simulink model "PubIfDecisionTOS_MDL"  (R2020b)
settings: configuration reference "DspaceConfig" (kept outside this file)
PostLoadFcn:
  | if any(exist('dsrtsu_mdlpostloadfcn', 'file') ~= 0), dsrtsu_mdlpostloadfcn('Execute', bdroot); end
InitFcn:
  | , if any(exist('dsmpb_private', 'file') ~= 0), dsmpb_private('dsmpb_mdlclblib', 'Init', bdroot); end,
undefined symbols (not defined in the file or in its folder): C_TOS_ACCEgoRAxletoFbumplength_m, C_TOS_ACCTargetFront_Flag, C_TOS_AEBJAPedObjDxThre_Val, C_TOS_AEBJAPedObjDyThre_Val, C_TOS_AEBJATargetSize_Val, C_TOS_AEBJAVehObjDxThre_Val, C_TOS_AEBJAVehObjDyThre_Val, C_TOS_AEBJuncPedTargetSize_Val, C_TOS_AEBLatObjDxThre_Val, C_TOS_AEBLatPedDyThre_Val, C_TOS_AEBLatTargetSize_Val, C_TOS_AEBLongTargetInEgoFront_Flag, C_TOS_axAbsGround_Parameter, C_TOS_CameraConfirmedFlag, C_TOS_CNsubjWidth, C_TOS_CurrentLaneCoreMinWidth_Val, C_TOS_CutInProb_Val_Zero, C_TOS_CutOutProb_Val_Zero, C_TOS_D2R_Val, C_TOS_DefaultValueObjectToCenterLine_dy, C_TOS_EgoCarWidth_Val, C_TOS_EgoDxRefPoint_m, C_TOS_EgoRAxletoFbumplength_m, C_TOS_HalfWidthVehicle_Con, C_TOS_HWA_CurrentLaneFlag, C_TOS_HWA_LeftLaneFlag, C_TOS_HWA_MovingDir_Vaild, C_TOS_HWA_MovState_Vaild, C_TOS_HWA_RightLaneFlag, C_TOS_LaneLineCourseErrorFront, C_TOS_LaneLineCourseErrorRear, C_TOS_MotorbikeDefaultWidth_m, C_TOS_NumberOfEffectiveTargets, C_TOS_Obj_Age_Val, C_TOS_Objdx_Constraint_Val, C_TOS_ObjectDefaultWidth_m, C_TOS_ObjInCurrentLane_Val, C_TOS_ObjInCurrentLaneValid, C_TOS_ObjInLeftLaneValid, C_TOS_ObjInRightLaneValid, C_TOS_ObjNotInCurrentLane_Val, C_TOS_ObjNotREElementType, C_TOS_ObjPredictDis_dy_ConstantVal_Zeros, C_TOS_ObjToCenterLine_ConstantVal_Zeros, C_TOS_OFMObjIDInvilad_Val, C_TOS_PIL_LatDisCons_Val_zero, C_TOS_PIL_ObjectCutInFlag_b, C_TOS_PIL_ObjectCutOutFlag_b, C_TOS_PIL_ObjLaneProb_al_Val, C_TOS_PP_ObjFusType_FC_Confirm_b, C_TOS_PP_ObjFusType_FC_FR_Confirm_b, C_TOS_PP_ObjFusType_FR_Confirm_b, C_TOS_RE_80BoolDefault_Val, C_TOS_RE_80Single181Default_Val, C_TOS_RE_80Single255Default_Val, C_TOS_RE_80Uint8Default_Val, C_TOS_RE_D2R, C_TOS_RE_D_180_Val, C_TOS_RE_InvalidObjectID_Val, C_TOS_RE_InvalidTargetChainDir_Val ... (+142)
libraries: simulink x1650, TOS_LIB x361, canfdmsglib x14
(part 58 of 69)

== system PubIfDecisionTOS_MDL/TOS_20201112/TOS_2012080320/TOS/AEB/TOS_AEBLong/AEBLong_Confirm/AEBLong/AEBLong_TrgConfirm/AEBLongTrgJudg/TOS_AEBLong_TargetMovingDir/ObjMovingDirSignalProcessing1/ObjMovingDirSignalProcessing2 ==
  note: fun2:目标运动方向处理 (ACC/AEB/HWA_LC/ELK/LCKie)
  PP_OncomingMovingDirFlg : Inport
  PP_CrossingMovingDirFlg : Inport  Port=2
  Object_MovingOrientation : Inport  Port=3
  Object_HeadingAngle : Inport  Port=4
  Abs : Abs
  Compare To Constant : simulink/Logic and Bit Operations/Compare To Constant  relop===  const=OFM_OBJ_ORIENTATION_E.NORTH  OutDataTypeStr=boolean
      settings: AttributesFormatString=OFM_OBJ_ORIENTATION_E.NORTH = 9
  Compare To Constant1 : simulink/Logic and Bit Operations/Compare To Constant  relop=>=  const=P_TOS_ObjInSameDirYawAngMinThre_Val  OutDataTypeStr=boolean
      settings: AttributesFormatString=P_TOS_ObjInSameDirYawAngMinThre_Val = 0
  Compare To Constant2 : simulink/Logic and Bit Operations/Compare To Constant  relop=<=  const=P_TOS_ObjInSameDirYawAngMaxThre_Val  OutDataTypeStr=boolean
      settings: AttributesFormatString=P_TOS_ObjInSameDirYawAngMaxThre_Val = 45
  Compare To Constant3 : simulink/Logic and Bit Operations/Compare To Constant  relop===  const=OFM_OBJ_ORIENTATION_E.SOUTH  OutDataTypeStr=boolean
      settings: AttributesFormatString=OFM_OBJ_ORIENTATION_E.SOUTH = 5
  Compare To Constant4 : simulink/Logic and Bit Operations/Compare To Constant  relop===  const=OFM_OBJ_ORIENTATION_E.WEST  OutDataTypeStr=boolean
      settings: AttributesFormatString=OFM_OBJ_ORIENTATION_E.WEST = 7
  Compare To Constant5 : simulink/Logic and Bit Operations/Compare To Constant  relop===  const=OFM_OBJ_ORIENTATION_E.EAST  OutDataTypeStr=boolean
      settings: AttributesFormatString=OFM_OBJ_ORIENTATION_E.EAST = 3
  Compare To Constant6 : simulink/Logic and Bit Operations/Compare To Constant  relop=>=  const=P_TOS_ObjLatCroYawAngMaxThre_Val  OutDataTypeStr=boolean
      settings: AttributesFormatString=P_TOS_ObjLatCroYawAngMaxThre_Val = 135
  Compare To Constant7 : simulink/Logic and Bit Operations/Compare To Constant  relop=<=  const=P_TOS_ObjOncomingYawAngMaxThre_Val  OutDataTypeStr=boolean
      settings: AttributesFormatString=P_TOS_ObjOncomingYawAngMaxThre_Val = 180
  Compare To Constant8 : simulink/Logic and Bit Operations/Compare To Constant  relop=>=  const=P_TOS_ObjLatCroYawAngMinThre_Val  OutDataTypeStr=boolean
      settings: AttributesFormatString=P_TOS_ObjLatCroYawAngMinThre_Val = 45
  Compare To Constant9 : simulink/Logic and Bit Operations/Compare To Constant  relop=<=  const=P_TOS_ObjLatCroYawAngMaxThre_Val  OutDataTypeStr=boolean
      settings: AttributesFormatString=P_TOS_ObjLatCroYawAngMaxThre_Val = 135
  Data Type Conversion1 : DataTypeConversion  OutDataTypeStr=uint8
  Data Type Conversion2 : DataTypeConversion  OutDataTypeStr=Enum: OFM_OBJ_ORIENTATION_E
  Enumerated Constant4 : simulink/Sources/Enumerated Constant  OutDataTypeStr=Enum: ObjectMovingOrientation_E  Value=ObjectMovingOrientation_E.SameDir  SampleTime=inf
      settings: AttributesFormatString=ObjectMovingOrientation_E.SameDir = 1
  Enumerated Constant5 : simulink/Sources/Enumerated Constant  OutDataTypeStr=Enum: ObjectMovingOrientation_E  Value=ObjectMovingOrientation_E.OnComingDir  SampleTime=inf
      settings: AttributesFormatString=ObjectMovingOrientation_E.OnComingDir = 2
  Enumerated Constant6 : simulink/Sources/Enumerated Constant  OutDataTypeStr=Enum: ObjectMovingOrientation_E  Value=ObjectMovingOrientation_E.Crossing  SampleTime=inf
      settings: AttributesFormatString=ObjectMovingOrientation_E.Crossing = 3
  Enumerated Constant7 : simulink/Sources/Enumerated Constant  OutDataTypeStr=Enum: ObjectMovingOrientation_E  Value=ObjectMovingOrientation_E.UnknownDir  SampleTime=inf
      settings: AttributesFormatString=ObjectMovingOrientation_E.UnknownDir = 0
  Logical Operator{7..10,13,15} (6 alike) : Logic  Operator=OR  AllPortsSameDT=off  OutDataTypeStr=boolean
  Logical Operator11 : Logic  AllPortsSameDT=off  OutDataTypeStr=boolean
  Logical Operator12 : Logic  AllPortsSameDT=off  OutDataTypeStr=boolean
  Logical Operator14 : Logic  AllPortsSameDT=off  OutDataTypeStr=boolean
  Switch3 : Switch  Criteria=u2 ~= 0
  Switch4 : Switch  Criteria=u2 ~= 0
  Switch5 : Switch  Criteria=u2 ~= 0
  PP_ObjMovingDirSignalProcessing : Outport
  wires:
  Data Type Conversion1/1 -> PP_ObjMovingDirSignalProcessing/1
  Object_MovingOrientation/1 -> Data Type Conversion2/1
  Object_HeadingAngle/1 -> Abs/1
  Logical Operator10/1 -> Logical Operator7/1
  PP_OncomingMovingDirFlg/1 -> [PP_OncomingMovingDirFlg]
  PP_CrossingMovingDirFlg/1 -> [PP_CrossingMovingDirFlg]
  [PP_OncomingMovingDirFlg] -> Logical Operator7/2
  [PP_CrossingMovingDirFlg] -> Logical Operator8/2
  Logical Operator14/1 -> Logical Operator13/2  "ObjLatCrossDirYawValid"
  Enumerated Constant6/1 -> Switch5/1
  Logical Operator12/1 -> Logical Operator9/2
  Compare To Constant6/1 -> Logical Operator11/1
  Compare To Constant1/1 -> Logical Operator12/1
  Enumerated Constant4/1 -> Switch3/1
  Logical Operator7/1 -> Switch4/2
  Logical Operator15/1 -> Logical Operator13/1
  Compare To Constant8/1 -> Logical Operator14/1
  Compare To Constant7/1 -> Logical Operator11/2
  Compare To Constant3/1 -> Logical Operator10/1
  Switch4/1 -> Switch5/3
  Logical Operator11/1 -> Logical Operator10/2
  Compare To Constant4/1 -> Logical Operator15/1
  Compare To Constant5/1 -> Logical Operator15/2
  Compare To Constant2/1 -> Logical Operator12/2
  Compare To Constant9/1 -> Logical Operator14/2
  Logical Operator9/1 -> Switch3/2
  Logical Operator8/1 -> Switch5/2
  Abs/1 -> Compare To Constant7/1, Compare To Constant1/1, Compare To Constant2/1, Compare To Constant6/1, Compare To Constant9/1, Compare To Constant8/1
  Enumerated Constant5/1 -> Switch4/1
  Enumerated Constant7/1 -> Switch3/3
  Compare To Constant/1 -> Logical Operator9/1
  Data Type Conversion2/1 -> Compare To Constant/1, Compare To Constant3/1, Compare To Constant5/1, Compare To Constant4/1
  Switch3/1 -> Switch4/3
  Logical Operator13/1 -> Logical Operator8/1
  Switch5/1 -> Data Type Conversion1/1

== system PubIfDecisionTOS_MDL/TOS_20201112/TOS_2012080320/TOS/AEB/TOS_AEBLong/AEBLong_Confirm/AEBLong/AEBLong_TrgConfirm/AEBLongTrgJudg/TOS_AEBLong_TargetMovingDir/ObjMovingDirSignalProcessing1/Oncoming_MovingDir_StrightLane ==
  Object_LM_PartInfor : Inport
  Bus Selector : BusSelector  OutputSignals=ObjectMappingVY
  Bus Selector1 : BusSelector  OutputSignals=ObjectMappingVX
  Bus Selector2 : BusSelector  OutputSignals=Object_DX
  Bus Selector3 : BusSelector  OutputSignals=Object_DY
  Bus Selector4 : BusSelector  OutputSignals=ObjectVYVXAngle
  Bus Selector5 : BusSelector  OutputSignals=Object_MovingState
  Compare To Constant : simulink/Logic and Bit Operations/Compare To Constant  relop===  const=OFM_OBJ_MOVINGSTATE_E.MOVING  OutDataTypeStr=boolean
  Data Type Conversion : DataTypeConversion  OutDataTypeStr=Enum: OFM_OBJ_MOVINGSTATE_E
  Logical Operator : Logic  AllPortsSameDT=off  OutDataTypeStr=boolean
  Logical Operator2 : Logic  AllPortsSameDT=off  OutDataTypeStr=boolean
  OncomingVXCondition : Subsystem
  OncomingVYCondition : Subsystem
  OncomingVYVXAngle : Subsystem
  Terminator : Terminator
  Terminator1 : Terminator
  PP_OncomingMovingDirFlg : Outport
  wires:
  Bus Selector1/1 -> OncomingVXCondition/1(Object_MappingVX), OncomingVYCondition/2(Object_MappingVX)  "<ObjectMappingVX>"
  Bus Selector/1 -> OncomingVYCondition/1(Object_MappingVY)  "<ObjectMappingVY>"
  OncomingVYCondition/1(OncomingVYflg) -> Logical Operator/1
  Bus Selector2/1 -> OncomingVXCondition/2(Object_DX)  "<Object_DX>"
  Bus Selector3/1 -> OncomingVXCondition/3(Object_DY)  "<Object_DY>"
  OncomingVXCondition/1(OncomingVXFlg) -> Logical Operator/2
  Object_LM_PartInfor/1 -> Bus Selector5/1, Bus Selector4/1, Bus Selector3/1, Bus Selector2/1, Bus Selector1/1, Bus Selector/1
  Bus Selector4/1 -> OncomingVYVXAngle/1(Object_VXVYAngle)  "<ObjectVYVXAngle>"
  Bus Selector5/1 -> Data Type Conversion/1  "<Object_MovingState>"
  Logical Operator/1 -> PP_OncomingMovingDirFlg/1
  Data Type Conversion/1 -> Compare To Constant/1
  Compare To Constant/1 -> Logical Operator2/1
  Logical Operator2/1 -> Terminator/1
  OncomingVYVXAngle/1(OncomingVYVXAngleFlg) -> Terminator1/1

== system PubIfDecisionTOS_MDL/TOS_20201112/TOS_2012080320/TOS/AEB/TOS_AEBLong/AEBLong_Confirm/AEBLong/AEBLong_TrgConfirm/AEBLongTrgJudg/TOS_AEBLong_TargetMovingDir/ObjMovingDirSignalProcessing1/Oncoming_MovingDir_StrightLane1 ==
  Object_LM_PartInfor : Inport
  Bus Selector : BusSelector  OutputSignals=ObjectMappingVX,ObjectMappingVY
  Bus Selector2 : BusSelector  OutputSignals=ObjectMappingVY,Object_DX,Object_DY
  Bus Selector4 : BusSelector  OutputSignals=ObjectVYVXAngle
  Bus Selector5 : BusSelector  OutputSignals=Object_MovingState
  Compare To Constant : simulink/Logic and Bit Operations/Compare To Constant  relop===  const=OFM_OBJ_MOVINGSTATE_E.MOVING  OutDataTypeStr=boolean
  CrossingVXCondition : Subsystem
  CrossingVYCondition : Subsystem
  CrossingVYVXAngle : Subsystem
  Data Type Conversion : DataTypeConversion  OutDataTypeStr=Enum: OFM_OBJ_MOVINGSTATE_E
  Logical Operator : Logic  AllPortsSameDT=off  OutDataTypeStr=boolean
  Logical Operator2 : Logic  AllPortsSameDT=off  OutDataTypeStr=boolean
  Terminator : Terminator
  Terminator1 : Terminator
  PP_CrossingMovingDirFlg : Outport
  wires:
  Bus Selector4/1 -> CrossingVYVXAngle/1(Object_VYVXAngle)  "<ObjectVYVXAngle>"
  CrossingVYCondition/1(CrossingVYFlg) -> Logical Operator/2
  Bus Selector2/2 -> CrossingVYCondition/2(Object_DX)  "<Object_DX>"
  CrossingVXCondition/1(CrossingVXflg) -> Logical Operator/1
  Bus Selector/1 -> CrossingVXCondition/1(Object_MappingVX)  "<ObjectMappingVX>"
  Bus Selector2/1 -> CrossingVYCondition/1(Object_MappingVY)  "<ObjectMappingVY>"
  Bus Selector2/3 -> CrossingVYCondition/3(Object_DY)  "<Object_DY>"
  Bus Selector/2 -> CrossingVXCondition/2(Object_MappingVY)  "<ObjectMappingVY>"
  Compare To Constant/1 -> Logical Operator2/1
  Object_LM_PartInfor/1 -> Bus Selector4/1, Bus Selector2/1, Bus Selector/1, Bus Selector5/1
  Bus Selector5/1 -> Data Type Conversion/1  "<Object_MovingState>"
  Data Type Conversion/1 -> Compare To Constant/1
  Logical Operator/1 -> PP_CrossingMovingDirFlg/1
  Logical Operator2/1 -> Terminator/1
  CrossingVYVXAngle/1(CrossingVYVXAngleFlg) -> Terminator1/1

== system PubIfDecisionTOS_MDL/TOS_20201112/TOS_2012080320/TOS/AEB/TOS_AEBLong/AEBLong_Confirm/AEBLong/AEBLong_TrgConfirm/AEBLongTrgJudg/TOS_AEBLong_TargetMovingDir/TOS_ACCMovingDirAborDly/If Action Subsystem ==
  TOS_AEBMovingDir : Inport
  Action Port : ActionPort  ActionPortLabel=else
  TOS_AEBMovingDirFilt : Outport
  wires:
  TOS_AEBMovingDir/1 -> TOS_AEBMovingDirFilt/1

== system PubIfDecisionTOS_MDL/TOS_20201112/TOS_2012080320/TOS/AEB/TOS_AEBLong/AEBLong_Confirm/AEBLong/AEBLong_TrgConfirm/AEBLongTrgJudg/TOS_AEBLong_TargetMovingDir/TOS_ACCMovingDirAborDly/If Action Subsystem1 ==
  TOS_AEBMovingDir : Inport
  Action Port : ActionPort  ActionPortLabel=if(u1)
  Constant : Constant  Value=0.15
  Constant4 : Constant  Value=0.05
  StateDelayAbortion : TOS_LIB/StateDelayAbortion  SystemSampleTime=-1  VariantActivationTime=update diagram  Latency=0  AutoFrameSizeCalculation=off
  TOS_AEBMovingDirFilt : Outport
  wires:
  TOS_AEBMovingDir/1 -> StateDelayAbortion/1
  Constant4/1 -> StateDelayAbortion/3
  Constant/1 -> StateDelayAbortion/2
  StateDelayAbortion/1 -> TOS_AEBMovingDirFilt/1

== system PubIfDecisionTOS_MDL/TOS_20201112/TOS_2012080320/TOS/AEB/TOS_AEBLong/AEBLong_Confirm/AEBLong/AEBLong_TrgConfirm/AEBLongTrgJudg/TOS_AEBLong_TargetMovingDir/TOS_ACCMovingDirAborDly/Subsystem ==
  AEBLong_Target_ID_K1 : Inport
  ObjectID : Inport  Port=2
  Relational Operator : RelationalOperator  Operator===  OutDataTypeStr=boolean  RndMeth=Simplest
  AEBLong_SameTargetP0 : Outport
  wires:
  AEBLong_Target_ID_K1/1 -> Relational Operator/1
  Relational Operator/1 -> AEBLong_SameTargetP0/1
  ObjectID/1 -> Relational Operator/2

== system PubIfDecisionTOS_MDL/TOS_20201112/TOS_2012080320/TOS/LC_LCKie_ELK/TOS_HWA/CurrentLane/HWA_CurrentLane_Target/HWA_CLF_Target_1/HWA_CLF_Target/HWA_CLF_Target/HWA_CLF_DyConfirm/OverLapConfirm ==
  DyConfirm_Sig : Inport
  Abs{,1..3} (4 alike) : Abs
  Add : Sum
  Bus Creator{1..4} (4 alike) : BusCreator  Inputs=2
  Bus Selector : BusSelector  OutputSignals=PositionFlag,Line_pC2
  Bus Selector1 : BusSelector  OutputSignals=PositionFlag,Line_pC2
  Bus Selector2 : BusSelector  OutputSignals=LM_LR_Line04_pC0,LM_RL_Line04_pC0
  Bus Selector3 : BusSelector  OutputSignals=PositionFlag,Line_pC2
  Bus Selector4 : BusSelector  OutputSignals=LM_LR_Line04_pC2,Object_DX,LM_LR_Line04_dDisStart,LM_LR_Line04_dDisEnd,LM_LR_Line04_fCamValid
  Bus Selector5 : BusSelector  OutputSignals=LM_LR_Line05_pC2,Object_DX,LM_LR_Line05_dDisStart,LM_LR_Line05_dDisEnd,LM_LR_Line05_fCamValid
  Bus Selector8 : BusSelector  OutputSignals=LM_LR_Line06_pC2,Object_DX,LM_LR_Line06_dDisStart,LM_LR_Line06_dDisEnd,LM_LR_Line06_fCamValid
  Compare To Constant : simulink/Logic and Bit Operations/Compare To Constant  relop===  const=uint8(4)  OutDataTypeStr=boolean
  Compare To Constant1 : simulink/Logic and Bit Operations/Compare To Constant  relop=>=  const=single(0.001)  OutDataTypeStr=boolean
  Compare To Constant2 : simulink/Logic and Bit Operations/Compare To Constant  relop=<=  const=single(0.1)  OutDataTypeStr=boolean
  Compare To Constant3 : simulink/Logic and Bit Operations/Compare To Constant  relop===  const=uint8(5)  OutDataTypeStr=boolean
  Compare To Constant4 : simulink/Logic and Bit Operations/Compare To Constant  relop=>=  const=single(0.001)  OutDataTypeStr=boolean
  Compare To Constant5 : simulink/Logic and Bit Operations/Compare To Constant  relop===  const=uint8(6)  OutDataTypeStr=boolean
  Compare To Constant6 : simulink/Logic and Bit Operations/Compare To Constant  relop=>=  const=single(0.001)  OutDataTypeStr=boolean
  Constant : Constant  Value=0  OutDataTypeStr=uint8
  Constant1 : Constant  Value=4  OutDataTypeStr=uint8
  Constant2 : Constant  Value=5  OutDataTypeStr=uint8
  Constant3 : Constant  Value=6  OutDataTypeStr=uint8
  Constant4 : Constant  Value=0  OutDataTypeStr=single
  Logical Operator1 : Logic  AllPortsSameDT=off  OutDataTypeStr=boolean
  Logical Operator10 : Logic  Inputs=3  AllPortsSameDT=off  OutDataTypeStr=boolean
  Logical Operator11 : Logic  Inputs=3  AllPortsSameDT=off  OutDataTypeStr=boolean
  Logical Operator2 : Logic  AllPortsSameDT=off  OutDataTypeStr=boolean
  Logical Operator3 : Logic  AllPortsSameDT=off  OutDataTypeStr=boolean
  Logical Operator4 : Logic  Operator=OR  Inputs=3  AllPortsSameDT=off  OutDataTypeStr=boolean
  Logical Operator5 : Logic  Operator=OR  AllPortsSameDT=off  OutDataTypeStr=boolean
  Logical Operator6 : Logic  Operator=OR  AllPortsSameDT=off  OutDataTypeStr=boolean
  Logical Operator7 : Logic  Operator=OR  AllPortsSameDT=off  OutDataTypeStr=boolean
  Logical Operator9 : Logic  Inputs=3  AllPortsSameDT=off  OutDataTypeStr=boolean
  Relational Operator4 : RelationalOperator  Operator=>  OutDataTypeStr=boolean  RndMeth=Simplest
  Relational Operator5 : RelationalOperator  Operator=<=  OutDataTypeStr=boolean  RndMeth=Simplest
  Relational Operator6 : RelationalOperator  Operator=>  OutDataTypeStr=boolean  RndMeth=Simplest
  Relational Operator7 : RelationalOperator  Operator=<=  OutDataTypeStr=boolean  RndMeth=Simplest
  Relational Operator8 : RelationalOperator  Operator=>  OutDataTypeStr=boolean  RndMeth=Simplest
  Relational Operator9 : RelationalOperator  Operator=<=  OutDataTypeStr=boolean  RndMeth=Simplest
  Signal Copy : SignalConversion  OverrideOpt=off
  Signal Copy1 : SignalConversion  OverrideOpt=off
  Signal Copy2 : SignalConversion  OverrideOpt=off
  Switch3 : Switch  Criteria=u2 > Threshold  OutDataTypeStr=single
  Switch4 : Switch  Criteria=u2 > Threshold  OutDataTypeStr=single
  Switch5 : Switch  Criteria=u2 > Threshold  OutDataTypeStr=single
  TOS_OverlapRatio : Outport
  wires:
  Abs3/1 -> Compare To Constant2/1
  Add/1 -> Abs3/1
  Logical Operator7/1 -> Logical Operator11/3
  [C0_Confirm] -> Logical Operator7/2
  Logical Operator6/1 -> Logical Operator10/3
  [C0_Confirm] -> Logical Operator6/2
  Logical Operator5/1 -> Logical Operator9/3
  [C0_Confirm] -> Logical Operator5/2
  Compare To Constant2/1 -> [C0_Confirm]
  Bus Selector2/2 -> Add/2  "<LM_RL_Line04_pC0>"
  Bus Selector2/1 -> Add/1  "<LM_LR_Line04_pC0>"
  Abs2/1 -> Compare To Constant6/1
  Abs1/1 -> Compare To Constant4/1
  Abs/1 -> Compare To Constant1/1
  Logical Operator4/1 -> TOS_OverlapRatio/1
  Logical Operator3/1 -> Logical Operator4/3
  Logical Operator2/1 -> Logical Operator4/2
  Bus Selector3/2 -> Abs2/1  "<Line_pC2>"
  Bus Selector3/1 -> Compare To Constant5/1  "<PositionFlag>"
  Switch3/1 -> Bus Selector/1, Bus Selector1/1, Bus Selector3/1
  Compare To Constant5/1 -> Logical Operator3/1
  Compare To Constant6/1 -> Logical Operator3/2
  Compare To Constant4/1 -> Logical Operator2/2
  Compare To Constant3/1 -> Logical Operator2/1
  Bus Selector1/1 -> Compare To Constant3/1  "<PositionFlag>"
  Bus Selector1/2 -> Abs1/1  "<Line_pC2>"
  Logical Operator1/1 -> Logical Operator4/1
  Compare To Constant1/1 -> Logical Operator1/2
  DyConfirm_Sig/1 -> Bus Selector2/1, Bus Selector4/1, Bus Selector5/1, Bus Selector8/1
  Compare To Constant/1 -> Logical Operator1/1
  Bus Selector/2 -> Abs/1  "<Line_pC2>"
  Bus Selector/1 -> Compare To Constant/1  "<PositionFlag>"
  Constant4/1 -> Bus Creator4/2  "Line_pC2"
  Bus Creator3/1 -> Switch5/1
  Signal Copy2/1 -> Bus Creator3/2  "Line_pC2"
  Bus Selector4/1 -> Signal Copy/1  "<LM_LR_Line04_pC2>"
  Logical Operator9/1 -> Switch3/2
  Bus Selector5/1 -> Signal Copy1/1  "<LM_LR_Line05_pC2>"
  Constant/1 -> Bus Creator4/1  "PositionFlag"
  Signal Copy1/1 -> Bus Creator2/2  "Line_pC2"
  Constant3/1 -> Bus Creator3/1  "PositionFlag"
  Constant2/1 -> Bus Creator2/1  "PositionFlag"
  Bus Selector4/4 -> Relational Operator5/2  "<LM_LR_Line04_dDisEnd>"
  Bus Creator4/1 -> Switch5/3
  Relational Operator7/1 -> Logical Operator10/2
  Relational Operator6/1 -> Logical Operator10/1
  Constant1/1 -> Bus Creator1/1  "PositionFlag"
  Relational Operator4/1 -> Logical Operator9/1
  Bus Creator2/1 -> Switch4/1
  Bus Selector5/5 -> Logical Operator6/1  "<LM_LR_Line05_fCamValid>"
  Switch5/1 -> Switch4/3
  Bus Selector8/5 -> Logical Operator7/1  "<LM_LR_Line06_fCamValid>"
  Bus Selector5/2 -> Relational Operator7/1, Relational Operator6/1  "<Object_DX>"
  Bus Selector5/3 -> Relational Operator6/2  "<LM_LR_Line05_dDisStart>"
  Logical Operator11/1 -> Switch5/2
  Bus Creator1/1 -> Switch3/1
  Bus Selector8/4 -> Relational Operator9/2  "<LM_LR_Line06_dDisEnd>"
  Switch4/1 -> Switch3/3
  Relational Operator9/1 -> Logical Operator11/2
  Bus Selector8/1 -> Signal Copy2/1  "<LM_LR_Line06_pC2>"
  Bus Selector8/3 -> Relational Operator8/2  "<LM_LR_Line06_dDisStart>"
  Signal Copy/1 -> Bus Creator1/2  "Line_pC2"
  Relational Operator5/1 -> Logical Operator9/2
  Relational Operator8/1 -> Logical Operator11/1
  Bus Selector4/2 -> Relational Operator4/1, Relational Operator5/1  "<Object_DX>"
  Bus Selector5/4 -> Relational Operator7/2  "<LM_LR_Line05_dDisEnd>"
  Bus Selector4/3 -> Relational Operator4/2  "<LM_LR_Line04_dDisStart>"
  Bus Selector4/5 -> Logical Operator5/1  "<LM_LR_Line04_fCamValid>"
  Bus Selector8/2 -> Relational Operator8/1, Relational Operator9/1  "<Object_DX>"
  Logical Operator10/1 -> Switch4/2

== system PubIfDecisionTOS_MDL/TOS_20201112/TOS_2012080320/TOS/LC_LCKie_ELK/TOS_HWA/CurrentLane/HWA_CurrentLane_Target/HWA_CLF_Target_1/HWA_CLF_Target/HWA_CLF_Target/HWA_CLF_FusionTypeConfirm/Subsystem1 ==
  ObjMovState : Inport
  HWA_CLF_Target_ID_K1 : Inport  Port=2
  HWA_CLF_Target_ID_K2 : Inport  Port=3
  HWA_CLF_Target_MovState_K1 : Inport  Port=4
  HWA_CLF_Target_MovState_K2 : Inport  Port=5
  ObjectID : Inport  Port=6
  TOS_ObjMovStateCfmFlow1 : Stateflow chart  TreatAsAtomicUnit=on
  TOS_ObjMovStateCfm : Outport
  wires:
  ObjectID/1 -> TOS_ObjMovStateCfmFlow1/6(ObjectID)
  ObjMovState/1 -> TOS_ObjMovStateCfmFlow1/5(ObjMovState)
  HWA_CLF_Target_MovState_K2/1 -> TOS_ObjMovStateCfmFlow1/4(Target_MovState_K2)
  HWA_CLF_Target_MovState_K1/1 -> TOS_ObjMovStateCfmFlow1/3(Target_MovState_K1)
  HWA_CLF_Target_ID_K2/1 -> TOS_ObjMovStateCfmFlow1/2(Target_ID_K2)
  HWA_CLF_Target_ID_K1/1 -> TOS_ObjMovStateCfmFlow1/1(Target_ID_K1)
  TOS_ObjMovStateCfmFlow1/1(TOS_ObjMovStateCfm) -> TOS_ObjMovStateCfm/1

== system PubIfDecisionTOS_MDL/TOS_20201112/TOS_2012080320/TOS/LC_LCKie_ELK/TOS_HWA/CurrentLane/HWA_CurrentLane_Target/HWA_CLF_Target_1/HWA_CLF_Target/HWA_CLF_Target/HWA_CLF_FusionTypeConfirm/TOS_ACCFusionTypeAborDly ==
  HWA_CLF_TargetP0_ID_K1 : Inport
  ObjectID : Inport  Port=2
  TOS_FusionType : Inport  Port=3
  If : If  IfExpression=u1
  If Action Subsystem : Subsystem  TreatAsAtomicUnit=on
  If Action Subsystem1 : Subsystem  TreatAsAtomicUnit=on
  Merge : Merge
  Relational Operator : RelationalOperator  Operator===  OutDataTypeStr=boolean  RndMeth=Simplest
  HWA_CLF_FusionTypeFilt : Outport
  wires:
  Merge/1 -> HWA_CLF_FusionTypeFilt/1
  If Action Subsystem/1(HWA_CLF_FusionTypeFilt) -> Merge/2
  If Action Subsystem1/1(HWA_CLF_FusionTypeFilt) -> Merge/1
  Relational Operator/1 -> If/1
  ObjectID/1 -> Relational Operator/2
  HWA_CLF_TargetP0_ID_K1/1 -> Relational Operator/1
  If/2 -> If Action Subsystem/Action
  TOS_FusionType/1 -> If Action Subsystem/1(HWA_CLF_FusionType), If Action Subsystem1/1(HWA_CLF_FusionType)
  If/1 -> If Action Subsystem1/Action

== system PubIfDecisionTOS_MDL/TOS_20201112/TOS_2012080320/TOS/LC_LCKie_ELK/TOS_HWA/CurrentLane/HWA_CurrentLane_Target/HWA_CLF_Target_1/HWA_CLF_Target/HWA_CLF_Target/HWA_CLF_ObjTypeConfirm/Subsystem ==
  ObjMovState : Inport
  Target_ID_K1 : Inport  Port=2
  Target_ID_K2 : Inport  Port=3
  Target_MovState_K1 : Inport  Port=4
  Target_MovState_K2 : Inport  Port=5
  ObjectID : Inport  Port=6
  TOS_ObjMovStateCfmFlow1 : Stateflow chart  TreatAsAtomicUnit=on
  TOS_ObjMovStateCfm : Outport
  wires:
  ObjectID/1 -> TOS_ObjMovStateCfmFlow1/6(ObjectID)
  ObjMovState/1 -> TOS_ObjMovStateCfmFlow1/5(ObjMovState)
  Target_MovState_K2/1 -> TOS_ObjMovStateCfmFlow1/4(ACC_TargetP0_MovState_K2)
  Target_MovState_K1/1 -> TOS_ObjMovStateCfmFlow1/3(ACC_TargetP0_MovState_K1)
  Target_ID_K2/1 -> TOS_ObjMovStateCfmFlow1/2(ACC_TargetP0_ID_K2)
  Target_ID_K1/1 -> TOS_ObjMovStateCfmFlow1/1(ACC_TargetP0_ID_K1)
  TOS_ObjMovStateCfmFlow1/1(TOS_ObjMovStateCfm) -> TOS_ObjMovStateCfm/1

== system PubIfDecisionTOS_MDL/TOS_20201112/TOS_2012080320/TOS/LC_LCKie_ELK/TOS_HWA/CurrentLane/HWA_CurrentLane_Target/HWA_CLF_Target_1/HWA_CLF_Target/HWA_CLF_Target/HWA_CLF_ObjTypeConfirm/TOS_ObjTypeAborDly ==
  Target_ID_K1 : Inport
  ObjectID : Inport  Port=2
  ObjType : Inport  Port=3
  If : If  IfExpression=u1
  If Action Subsystem : Subsystem  TreatAsAtomicUnit=on
  If Action Subsystem1 : Subsystem  TreatAsAtomicUnit=on
  Merge : Merge
  Relational Operator : RelationalOperator  Operator===  OutDataTypeStr=boolean  RndMeth=Simplest
  ObjTypeFilt : Outport
  wires:
  Merge/1 -> ObjTypeFilt/1
  If Action Subsystem/1(FusionTypeFilt) -> Merge/2
  If Action Subsystem1/1(FusionTypeFilt) -> Merge/1
  Relational Operator/1 -> If/1
  ObjectID/1 -> Relational Operator/2
  Target_ID_K1/1 -> Relational Operator/1
  If/2 -> If Action Subsystem/Action
  ObjType/1 -> If Action Subsystem/1(FusionType), If Action Subsystem1/1(FusionType)
  If/1 -> If Action Subsystem1/Action

== system PubIfDecisionTOS_MDL/TOS_20201112/TOS_2012080320/TOS/LC_LCKie_ELK/TOS_HWA/CurrentLane/HWA_CurrentLane_Target/HWA_CLF_Target_1/HWA_CLF_Target/HWA_CLF_Target/HWA_CLF_ObstacleProbConfirm/ObstacleProbAborDly ==
  Target_ID_K1 : Inport
  ObjectID : Inport  Port=2
  ObstacleProb : Inport  Port=3
  If : If  IfExpression=u1
  If Action Subsystem : Subsystem  TreatAsAtomicUnit=on
  If Action Subsystem1 : Subsystem  TreatAsAtomicUnit=on
  Merge : Merge
  Subsystem : Subsystem
  ObstacleProbFilt : Outport
  wires:
  Merge/1 -> ObstacleProbFilt/1
  If Action Subsystem/1(FusionTypeFilt) -> Merge/2
  If Action Subsystem1/1(FusionTypeFilt) -> Merge/1
  Subsystem/1(SameTargetP0) -> If/1
  ObjectID/1 -> Subsystem/2(ObjectID)
  Target_ID_K1/1 -> Subsystem/1(TargetP0_ID_K1)
  If/2 -> If Action Subsystem/Action
  ObstacleProb/1 -> If Action Subsystem/1(FusionType), If Action Subsystem1/1(FusionType)
  If/1 -> If Action Subsystem1/Action

== system PubIfDecisionTOS_MDL/TOS_20201112/TOS_2012080320/TOS/LC_LCKie_ELK/TOS_HWA/CurrentLane/HWA_CurrentLane_Target/HWA_CLF_Target_1/HWA_CLF_Target/HWA_CLF_Target/HWA_CLF_TargetMovingDirConfirm/HWA_MovingDirAborDly ==
  HWA_TargetP0_ID_K1 : Inport
  ObjectID : Inport  Port=2
  HWA_MovingDir : Inport  Port=3
  If : If  IfExpression=u1
  If Action Subsystem : Subsystem  TreatAsAtomicUnit=on
  If Action Subsystem1 : Subsystem  TreatAsAtomicUnit=on
  Merge : Merge
  Subsystem : Subsystem
  HWA_TrgMovDirFlag_6_ObserVale : Outport
  HWA_TrgMovDir : Outport  Port=2
  wires:
  Merge/1 -> HWA_TrgMovDir/1
  If Action Subsystem/1(TOS_MovingDirFilt) -> Merge/2
  If Action Subsystem1/1(TOS_MovingDirFilt) -> Merge/1
  Subsystem/1(ACC_SameTargetP0) -> If/1, HWA_TrgMovDirFlag_6_ObserVale/1
  ObjectID/1 -> Subsystem/2(ObjectID)
  HWA_TargetP0_ID_K1/1 -> Subsystem/1(ACC_TargetP0_ID_K1)
  If/2 -> If Action Subsystem/Action
  HWA_MovingDir/1 -> If Action Subsystem/1(TOS_MovingDir), If Action Subsystem1/1(TOS_MovingDir)
  If/1 -> If Action Subsystem1/Action

== system PubIfDecisionTOS_MDL/TOS_20201112/TOS_2012080320/TOS/LC_LCKie_ELK/TOS_HWA/CurrentLane/HWA_CurrentLane_Target/HWA_CLF_Target_1/HWA_CLF_Target/HWA_CLF_Target/HWA_CLF_TargetMovingDirConfirm/Subsystem ==
  ObjMovState : Inport
  ACC_Target_ID_K1 : Inport  Port=2
  ACC_Target_ID_K2 : Inport  Port=3
  ACC_Target_MovState_K1 : Inport  Port=4
  ACC_Target_MovState_K2 : Inport  Port=5
  ObjectID : Inport  Port=6
  TOS_ObjMovStateCfmFlow : Stateflow chart  TreatAsAtomicUnit=on
  TOS_ObjMovStateCfm : Outport
  wires:
  ObjectID/1 -> TOS_ObjMovStateCfmFlow/6(ObjectID)
  ObjMovState/1 -> TOS_ObjMovStateCfmFlow/5(ObjMovState)
  ACC_Target_MovState_K2/1 -> TOS_ObjMovStateCfmFlow/4(Target_MovState_K2)
  ACC_Target_MovState_K1/1 -> TOS_ObjMovStateCfmFlow/3(Target_MovState_K1)
  ACC_Target_ID_K2/1 -> TOS_ObjMovStateCfmFlow/2(Target_ID_K2)
  ACC_Target_ID_K1/1 -> TOS_ObjMovStateCfmFlow/1(Target_ID_K1)
  TOS_ObjMovStateCfmFlow/1(TOS_ObjMovStateCfm) -> TOS_ObjMovStateCfm/1

== system PubIfDecisionTOS_MDL/TOS_20201112/TOS_2012080320/TOS/LC_LCKie_ELK/TOS_HWA/CurrentLane/HWA_CurrentLane_Target/HWA_CLF_Target_2/HWA_CLF_Target/HWA_CLF_Target/HWA_CLF_DyConfirm/OverLapConfirm ==
  note: 0.00125
  DyConfirm_Sig : Inport
  Abs{,1..3} (4 alike) : Abs
  Add : Sum
  Bus Creator{1..4} (4 alike) : BusCreator  Inputs=2
  Bus Selector : BusSelector  OutputSignals=PositionFlag,Line_pC2
  Bus Selector1 : BusSelector  OutputSignals=PositionFlag,Line_pC2
  Bus Selector2 : BusSelector  OutputSignals=LM_LR_Line04_pC0,LM_RL_Line04_pC0
  Bus Selector3 : BusSelector  OutputSignals=PositionFlag,Line_pC2
  Bus Selector4 : BusSelector  OutputSignals=LM_LR_Line04_pC2,Object_DX,LM_LR_Line04_dDisStart,LM_LR_Line04_dDisEnd,LM_LR_Line04_fCamValid
  Bus Selector5 : BusSelector  OutputSignals=LM_LR_Line05_pC2,Object_DX,LM_LR_Line05_dDisStart,LM_LR_Line05_dDisEnd,LM_LR_Line05_fCamValid
  Bus Selector8 : BusSelector  OutputSignals=LM_LR_Line06_pC2,Object_DX,LM_LR_Line06_dDisStart,LM_LR_Line06_dDisEnd,LM_LR_Line06_fCamValid
  Compare To Constant : simulink/Logic and Bit Operations/Compare To Constant  relop===  const=uint8(4)  OutDataTypeStr=boolean
  Compare To Constant1 : simulink/Logic and Bit Operations/Compare To Constant  relop=>=  const=single(0.001)  OutDataTypeStr=boolean
  Compare To Constant2 : simulink/Logic and Bit Operations/Compare To Constant  relop=<=  const=single(0.1)  OutDataTypeStr=boolean
  Compare To Constant3 : simulink/Logic and Bit Operations/Compare To Constant  relop===  const=uint8(5)  OutDataTypeStr=boolean
  Compare To Constant4 : simulink/Logic and Bit Operations/Compare To Constant  relop=>=  const=single(0.001)  OutDataTypeStr=boolean
  Compare To Constant5 : simulink/Logic and Bit Operations/Compare To Constant  relop===  const=uint8(6)  OutDataTypeStr=boolean
  Compare To Constant6 : simulink/Logic and Bit Operations/Compare To Constant  relop=>=  const=single(0.001)  OutDataTypeStr=boolean
  Constant : Constant  Value=0  OutDataTypeStr=uint8
  Constant1 : Constant  Value=4  OutDataTypeStr=uint8
  Constant2 : Constant  Value=5  OutDataTypeStr=uint8
  Constant3 : Constant  Value=6  OutDataTypeStr=uint8
  Constant4 : Constant  Value=0  OutDataTypeStr=single
  Logical Operator1 : Logic  AllPortsSameDT=off  OutDataTypeStr=boolean
  Logical Operator10 : Logic  Inputs=3  AllPortsSameDT=off  OutDataTypeStr=boolean
  Logical Operator11 : Logic  Inputs=3  AllPortsSameDT=off  OutDataTypeStr=boolean
  Logical Operator2 : Logic  AllPortsSameDT=off  OutDataTypeStr=boolean
  Logical Operator3 : Logic  AllPortsSameDT=off  OutDataTypeStr=boolean
  Logical Operator4 : Logic  Operator=OR  Inputs=3  AllPortsSameDT=off  OutDataTypeStr=boolean
  Logical Operator5 : Logic  Operator=OR  AllPortsSameDT=off  OutDataTypeStr=boolean
  Logical Operator6 : Logic  Operator=OR  AllPortsSameDT=off  OutDataTypeStr=boolean
  Logical Operator7 : Logic  Operator=OR  AllPortsSameDT=off  OutDataTypeStr=boolean
  Logical Operator9 : Logic  Inputs=3  AllPortsSameDT=off  OutDataTypeStr=boolean
  Relational Operator4 : RelationalOperator  Operator=>  OutDataTypeStr=boolean  RndMeth=Simplest
  Relational Operator5 : RelationalOperator  Operator=<=  OutDataTypeStr=boolean  RndMeth=Simplest
  Relational Operator6 : RelationalOperator  Operator=>  OutDataTypeStr=boolean  RndMeth=Simplest
  Relational Operator7 : RelationalOperator  Operator=<=  OutDataTypeStr=boolean  RndMeth=Simplest
  Relational Operator8 : RelationalOperator  Operator=>  OutDataTypeStr=boolean  RndMeth=Simplest
  Relational Operator9 : RelationalOperator  Operator=<=  OutDataTypeStr=boolean  RndMeth=Simplest
  Signal Copy : SignalConversion  OverrideOpt=off
  Signal Copy1 : SignalConversion  OverrideOpt=off
  Signal Copy2 : SignalConversion  OverrideOpt=off
  Switch3 : Switch  Criteria=u2 > Threshold  OutDataTypeStr=single
  Switch4 : Switch  Criteria=u2 > Threshold  OutDataTypeStr=single
  Switch5 : Switch  Criteria=u2 > Threshold  OutDataTypeStr=single
  TOS_OverlapRatio : Outport
  wires:
  Logical Operator10/1 -> Switch4/2
  Bus Selector8/2 -> Relational Operator9/1, Relational Operator8/1  "<Object_DX>"
  Bus Selector4/5 -> Logical Operator5/1  "<LM_LR_Line04_fCamValid>"
  Bus Selector4/3 -> Relational Operator4/2  "<LM_LR_Line04_dDisStart>"
  Bus Selector5/4 -> Relational Operator7/2  "<LM_LR_Line05_dDisEnd>"
  Bus Selector4/2 -> Relational Operator5/1, Relational Operator4/1  "<Object_DX>"
  Relational Operator8/1 -> Logical Operator11/1
  Relational Operator5/1 -> Logical Operator9/2
  Signal Copy/1 -> Bus Creator1/2  "Line_pC2"
  Bus Selector8/3 -> Relational Operator8/2  "<LM_LR_Line06_dDisStart>"
  Bus Selector8/1 -> Signal Copy2/1  "<LM_LR_Line06_pC2>"
  Relational Operator9/1 -> Logical Operator11/2
  Switch4/1 -> Switch3/3
  Bus Selector8/4 -> Relational Operator9/2  "<LM_LR_Line06_dDisEnd>"
  Bus Creator1/1 -> Switch3/1
  Logical Operator11/1 -> Switch5/2
  Bus Selector5/3 -> Relational Operator6/2  "<LM_LR_Line05_dDisStart>"
  Bus Selector5/2 -> Relational Operator6/1, Relational Operator7/1  "<Object_DX>"
  Bus Selector8/5 -> Logical Operator7/1  "<LM_LR_Line06_fCamValid>"
  Switch5/1 -> Switch4/3
  Bus Selector5/5 -> Logical Operator6/1  "<LM_LR_Line05_fCamValid>"
  Bus Creator2/1 -> Switch4/1
  Relational Operator4/1 -> Logical Operator9/1
  Constant1/1 -> Bus Creator1/1  "PositionFlag"
  Relational Operator6/1 -> Logical Operator10/1
  Relational Operator7/1 -> Logical Operator10/2
  Bus Creator4/1 -> Switch5/3
  Bus Selector4/4 -> Relational Operator5/2  "<LM_LR_Line04_dDisEnd>"
  Constant2/1 -> Bus Creator2/1  "PositionFlag"
  Constant3/1 -> Bus Creator3/1  "PositionFlag"
  Signal Copy1/1 -> Bus Creator2/2  "Line_pC2"
  Constant/1 -> Bus Creator4/1  "PositionFlag"
  Bus Selector5/1 -> Signal Copy1/1  "<LM_LR_Line05_pC2>"
  Logical Operator9/1 -> Switch3/2
  Bus Selector4/1 -> Signal Copy/1  "<LM_LR_Line04_pC2>"
  Signal Copy2/1 -> Bus Creator3/2  "Line_pC2"
  Bus Creator3/1 -> Switch5/1
  Constant4/1 -> Bus Creator4/2  "Line_pC2"
  Bus Selector/1 -> Compare To Constant/1  "<PositionFlag>"
  Bus Selector/2 -> Abs/1  "<Line_pC2>"
  Compare To Constant/1 -> Logical Operator1/1
  DyConfirm_Sig/1 -> Bus Selector8/1, Bus Selector5/1, Bus Selector4/1, Bus Selector2/1
  Compare To Constant1/1 -> Logical Operator1/2
  Logical Operator1/1 -> Logical Operator4/1
  Bus Selector1/2 -> Abs1/1  "<Line_pC2>"
  Bus Selector1/1 -> Compare To Constant3/1  "<PositionFlag>"
  Compare To Constant3/1 -> Logical Operator2/1
  Compare To Constant4/1 -> Logical Operator2/2
  Compare To Constant6/1 -> Logical Operator3/2
  Compare To Constant5/1 -> Logical Operator3/1
  Switch3/1 -> Bus Selector3/1, Bus Selector1/1, Bus Selector/1
  Bus Selector3/1 -> Compare To Constant5/1  "<PositionFlag>"
  Bus Selector3/2 -> Abs2/1  "<Line_pC2>"
  Logical Operator2/1 -> Logical Operator4/2
  Logical Operator3/1 -> Logical Operator4/3
  Logical Operator4/1 -> TOS_OverlapRatio/1
  Abs/1 -> Compare To Constant1/1
  Abs1/1 -> Compare To Constant4/1
  Abs2/1 -> Compare To Constant6/1
  Bus Selector2/1 -> Add/1  "<LM_LR_Line04_pC0>"
  Bus Selector2/2 -> Add/2  "<LM_RL_Line04_pC0>"
  Compare To Constant2/1 -> [C0_Confirm]
  [C0_Confirm] -> Logical Operator5/2
  Logical Operator5/1 -> Logical Operator9/3
  [C0_Confirm] -> Logical Operator6/2
  Logical Operator6/1 -> Logical Operator10/3
  [C0_Confirm] -> Logical Operator7/2
  Logical Operator7/1 -> Logical Operator11/3
  Add/1 -> Abs3/1
  Abs3/1 -> Compare To Constant2/1

== system PubIfDecisionTOS_MDL/TOS_20201112/TOS_2012080320/TOS/LC_LCKie_ELK/TOS_HWA/CurrentLane/HWA_CurrentLane_Target/HWA_CLF_Target_2/HWA_CLF_Target/HWA_CLF_Target/HWA_CLF_FusionTypeConfirm/Subsystem1 ==
  ObjMovState : Inport
  HWA_CLF_Target_ID_K1 : Inport  Port=2
  HWA_CLF_Target_ID_K2 : Inport  Port=3
  HWA_CLF_Target_MovState_K1 : Inport  Port=4
  HWA_CLF_Target_MovState_K2 : Inport  Port=5
  ObjectID : Inport  Port=6
  TOS_ObjMovStateCfmFlow1 : Stateflow chart  TreatAsAtomicUnit=on
  TOS_ObjMovStateCfm : Outport
  wires:
  TOS_ObjMovStateCfmFlow1/1(TOS_ObjMovStateCfm) -> TOS_ObjMovStateCfm/1
  HWA_CLF_Target_ID_K1/1 -> TOS_ObjMovStateCfmFlow1/1(Target_ID_K1)
  HWA_CLF_Target_ID_K2/1 -> TOS_ObjMovStateCfmFlow1/2(Target_ID_K2)
  HWA_CLF_Target_MovState_K1/1 -> TOS_ObjMovStateCfmFlow1/3(Target_MovState_K1)
  HWA_CLF_Target_MovState_K2/1 -> TOS_ObjMovStateCfmFlow1/4(Target_MovState_K2)
  ObjMovState/1 -> TOS_ObjMovStateCfmFlow1/5(ObjMovState)
  ObjectID/1 -> TOS_ObjMovStateCfmFlow1/6(ObjectID)

== system PubIfDecisionTOS_MDL/TOS_20201112/TOS_2012080320/TOS/LC_LCKie_ELK/TOS_HWA/CurrentLane/HWA_CurrentLane_Target/HWA_CLF_Target_2/HWA_CLF_Target/HWA_CLF_Target/HWA_CLF_FusionTypeConfirm/TOS_ACCFusionTypeAborDly ==
  HWA_CLF_TargetP0_ID_K1 : Inport
  ObjectID : Inport  Port=2
  TOS_FusionType : Inport  Port=3
  If : If  IfExpression=u1
  If Action Subsystem : Subsystem  TreatAsAtomicUnit=on
  If Action Subsystem1 : Subsystem  TreatAsAtomicUnit=on
  Merge : Merge
  Relational Operator : RelationalOperator  Operator===  OutDataTypeStr=boolean  RndMeth=Simplest
  HWA_CLF_FusionTypeFilt : Outport
  wires:
  If/1 -> If Action Subsystem1/Action
  TOS_FusionType/1 -> If Action Subsystem1/1(HWA_CLF_FusionType), If Action Subsystem/1(HWA_CLF_FusionType)
  If/2 -> If Action Subsystem/Action
  HWA_CLF_TargetP0_ID_K1/1 -> Relational Operator/1
  ObjectID/1 -> Relational Operator/2
  Relational Operator/1 -> If/1
  If Action Subsystem1/1(HWA_CLF_FusionTypeFilt) -> Merge/1
  If Action Subsystem/1(HWA_CLF_FusionTypeFilt) -> Merge/2
  Merge/1 -> HWA_CLF_FusionTypeFilt/1

== system PubIfDecisionTOS_MDL/TOS_20201112/TOS_2012080320/TOS/LC_LCKie_ELK/TOS_HWA/CurrentLane/HWA_CurrentLane_Target/HWA_CLF_Target_2/HWA_CLF_Target/HWA_CLF_Target/HWA_CLF_ObjTypeConfirm/Subsystem ==
  ObjMovState : Inport
  Target_ID_K1 : Inport  Port=2
  Target_ID_K2 : Inport  Port=3
  Target_MovState_K1 : Inport  Port=4
  Target_MovState_K2 : Inport  Port=5
  ObjectID : Inport  Port=6
  TOS_ObjMovStateCfmFlow1 : Stateflow chart  TreatAsAtomicUnit=on
  TOS_ObjMovStateCfm : Outport
  wires:
  TOS_ObjMovStateCfmFlow1/1(TOS_ObjMovStateCfm) -> TOS_ObjMovStateCfm/1
  Target_ID_K1/1 -> TOS_ObjMovStateCfmFlow1/1(ACC_TargetP0_ID_K1)
  Target_ID_K2/1 -> TOS_ObjMovStateCfmFlow1/2(ACC_TargetP0_ID_K2)
  Target_MovState_K1/1 -> TOS_ObjMovStateCfmFlow1/3(ACC_TargetP0_MovState_K1)
  Target_MovState_K2/1 -> TOS_ObjMovStateCfmFlow1/4(ACC_TargetP0_MovState_K2)
  ObjMovState/1 -> TOS_ObjMovStateCfmFlow1/5(ObjMovState)
  ObjectID/1 -> TOS_ObjMovStateCfmFlow1/6(ObjectID)

== system PubIfDecisionTOS_MDL/TOS_20201112/TOS_2012080320/TOS/LC_LCKie_ELK/TOS_HWA/CurrentLane/HWA_CurrentLane_Target/HWA_CLF_Target_2/HWA_CLF_Target/HWA_CLF_Target/HWA_CLF_ObjTypeConfirm/TOS_ObjTypeAborDly ==
  Target_ID_K1 : Inport
  ObjectID : Inport  Port=2
  ObjType : Inport  Port=3
  If : If  IfExpression=u1
  If Action Subsystem : Subsystem  TreatAsAtomicUnit=on
  If Action Subsystem1 : Subsystem  TreatAsAtomicUnit=on
  Merge : Merge
  Relational Operator : RelationalOperator  Operator===  OutDataTypeStr=boolean  RndMeth=Simplest
  ObjTypeFilt : Outport
  wires:
  If/1 -> If Action Subsystem1/Action
  ObjType/1 -> If Action Subsystem1/1(FusionType), If Action Subsystem/1(FusionType)
  If/2 -> If Action Subsystem/Action
  Target_ID_K1/1 -> Relational Operator/1
  ObjectID/1 -> Relational Operator/2
  Relational Operator/1 -> If/1
  If Action Subsystem1/1(FusionTypeFilt) -> Merge/1
  If Action Subsystem/1(FusionTypeFilt) -> Merge/2
  Merge/1 -> ObjTypeFilt/1

== system PubIfDecisionTOS_MDL/TOS_20201112/TOS_2012080320/TOS/LC_LCKie_ELK/TOS_HWA/CurrentLane/HWA_CurrentLane_Target/HWA_CLF_Target_2/HWA_CLF_Target/HWA_CLF_Target/HWA_CLF_ObstacleProbConfirm/ObstacleProbAborDly ==
  Target_ID_K1 : Inport
  ObjectID : Inport  Port=2
  ObstacleProb : Inport  Port=3
  If : If  IfExpression=u1
  If Action Subsystem : Subsystem  TreatAsAtomicUnit=on
  If Action Subsystem1 : Subsystem  TreatAsAtomicUnit=on
  Merge : Merge
  Subsystem : Subsystem
  ObstacleProbFilt : Outport
  wires:
  If/1 -> If Action Subsystem1/Action
  ObstacleProb/1 -> If Action Subsystem1/1(FusionType), If Action Subsystem/1(FusionType)
  If/2 -> If Action Subsystem/Action
  Target_ID_K1/1 -> Subsystem/1(TargetP0_ID_K1)
  ObjectID/1 -> Subsystem/2(ObjectID)
  Subsystem/1(SameTargetP0) -> If/1
  If Action Subsystem1/1(FusionTypeFilt) -> Merge/1
  If Action Subsystem/1(FusionTypeFilt) -> Merge/2
  Merge/1 -> ObstacleProbFilt/1

== system PubIfDecisionTOS_MDL/TOS_20201112/TOS_2012080320/TOS/LC_LCKie_ELK/TOS_HWA/CurrentLane/HWA_CurrentLane_Target/HWA_CLF_Target_2/HWA_CLF_Target/HWA_CLF_Target/HWA_CLF_TargetMovingDirConfirm/HWA_MovingDirAborDly ==
  HWA_TargetP0_ID_K1 : Inport
  ObjectID : Inport  Port=2
  HWA_MovingDir : Inport  Port=3
  If : If  IfExpression=u1
  If Action Subsystem : Subsystem  TreatAsAtomicUnit=on
  If Action Subsystem1 : Subsystem  TreatAsAtomicUnit=on
  Merge : Merge
  Subsystem : Subsystem
  HWA_TrgMovDirFlag_6_ObserVale : Outport
  HWA_TrgMovDir : Outport  Port=2
  wires:
  If/1 -> If Action Subsystem1/Action
  HWA_MovingDir/1 -> If Action Subsystem1/1(TOS_MovingDir), If Action Subsystem/1(TOS_MovingDir)
  If/2 -> If Action Subsystem/Action
  HWA_TargetP0_ID_K1/1 -> Subsystem/1(ACC_TargetP0_ID_K1)
  ObjectID/1 -> Subsystem/2(ObjectID)
  Subsystem/1(ACC_SameTargetP0) -> HWA_TrgMovDirFlag_6_ObserVale/1, If/1
  If Action Subsystem1/1(TOS_MovingDirFilt) -> Merge/1
  If Action Subsystem/1(TOS_MovingDirFilt) -> Merge/2
  Merge/1 -> HWA_TrgMovDir/1

== system PubIfDecisionTOS_MDL/TOS_20201112/TOS_2012080320/TOS/LC_LCKie_ELK/TOS_HWA/CurrentLane/HWA_CurrentLane_Target/HWA_CLF_Target_2/HWA_CLF_Target/HWA_CLF_Target/HWA_CLF_TargetMovingDirConfirm/Subsystem ==
  ObjMovState : Inport
  ACC_Target_ID_K1 : Inport  Port=2
  ACC_Target_ID_K2 : Inport  Port=3
  ACC_Target_MovState_K1 : Inport  Port=4
  ACC_Target_MovState_K2 : Inport  Port=5
  ObjectID : Inport  Port=6
  TOS_ObjMovStateCfmFlow : Stateflow chart  TreatAsAtomicUnit=on
  TOS_ObjMovStateCfm : Outport
  wires:
  TOS_ObjMovStateCfmFlow/1(TOS_ObjMovStateCfm) -> TOS_ObjMovStateCfm/1
  ACC_Target_ID_K1/1 -> TOS_ObjMovStateCfmFlow/1(Target_ID_K1)
  ACC_Target_ID_K2/1 -> TOS_ObjMovStateCfmFlow/2(Target_ID_K2)
  ACC_Target_MovState_K1/1 -> TOS_ObjMovStateCfmFlow/3(Target_MovState_K1)
  ACC_Target_MovState_K2/1 -> TOS_ObjMovStateCfmFlow/4(Target_MovState_K2)
  ObjMovState/1 -> TOS_ObjMovStateCfmFlow/5(ObjMovState)
  ObjectID/1 -> TOS_ObjMovStateCfmFlow/6(ObjectID)
